simulink model "Control_scheme"  (R2020b)
settings: Solver=VariableStepAuto  StartTime=0.0  StopTime=200  RelTol=1e-3
values from neighbouring files (symbols this model uses):
  A = [5.11995503588 1 0 0 0 0 -11.4260465467 0 1 0 0 0 ... (36 elements, 6x6)]    [Estimated_Model.mat]
  Atrue = [-232280.917083 -1161395.21042 -696840.50125 -929117.855833 -232280.917083 -116142.271042 -247175.760189 -1235880.44867 -741527.985114 -988703.898712 -247175.851098 -123588.02214 ... (36 elements, 6x6)]    [barrassmodel2.mat]
  B = [1 0 0 0 0 0]    [Estimated_Model.mat]
  Btrue = [1 5 3 4 1 0.5]    [barrassmodel2.mat]
  C = [-6.48338492424e-05 0.00041393325507 -0.000527701144131 0.00055117489166 -0.000426728644373 0]    [Estimated_Model.mat]
  Ctrue = [2750000 -2204545.45455 32477272.7273 -15227272.7273 -18704545.4545 -19090909.0909]    [barrassmodel2.mat]
  D = 0    [Estimated_Model.mat]
  Dtrue = 0    [barrassmodel2.mat]
  Nbar = Nu+K*Nx    [LQE_LQR_par.m]    (also in demo.m)
  Ts = 1/fs    (= 0.01)    [BasicSim.m]    (also in IdentificationAlgorithm_best.m; LQE_LQR_par.m; demo.m)
undefined symbols (not defined in the file or in its folder): DiscIntNeverNeededParam, K, M
libraries: simulink x8
settings Model: Creator=Tripaskio  LastModifiedBy=renato

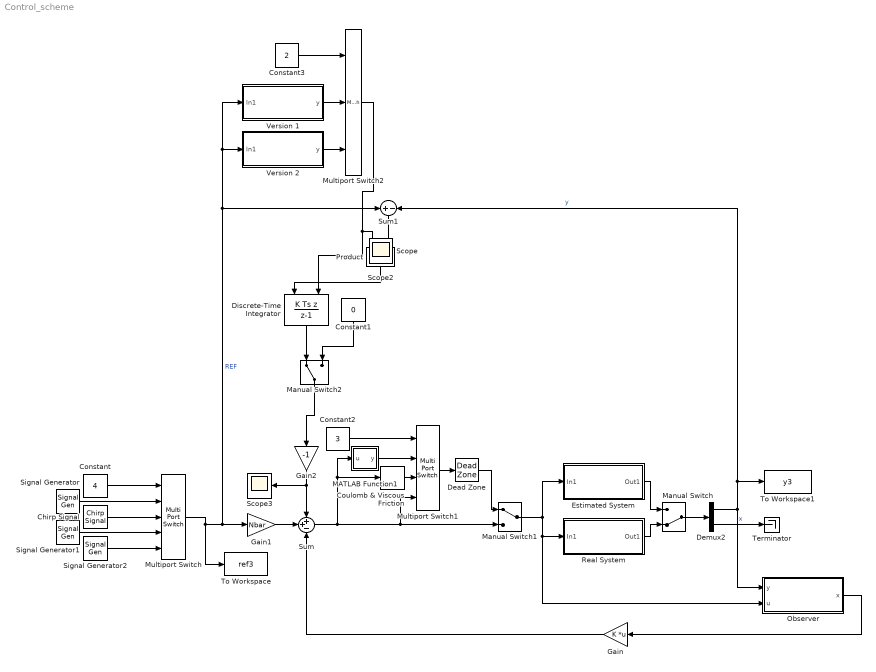
== system Control_scheme ==
  Chirp Signal : simulink/Sources/Chirp Signal  f1=0.01  T=200  f2=0.1
  Constant : Constant  Value=4
  Constant1 : Constant  Value=0
  Constant2 : Constant  Value=3
  Constant3 : Constant  Value=2
  Coulomb & Viscous Friction : simulink/Discontinuities/Coulomb & Viscous Friction  offset=[0.1]  gain=1
  Dead Zone : DeadZone  LowerValue=-0.1  UpperValue=0.1  SaturateOnIntegerOverflow=on
  Demux2 : Demux  Outputs=[1,6]
  Discrete-Time Integrator : DiscreteIntegrator  IntegratorMethod=Integration: Backward Euler  gainval=0.011  ExternalReset=either  SampleTime=-1  UpperSaturationLimit=10  LowerSaturationLimit=-10  ICPrevOutput=DiscIntNeverNeededParam  ICPrevScaledInput=DiscIntNeverNeededParam
  Estimated System : Subsystem
  Gain : Gain  Gain=K  Multiplication=Matrix(K*u)
  Gain1 : Gain  Gain=Nbar
  Gain2 : Gain  Gain=-1
  MATLAB Function1 : MATLAB Function  TreatAsAtomicUnit=on
  Manual Switch : ManualSwitch  CurrentSetting=0
  Manual Switch1 : ManualSwitch
  Manual Switch2 : ManualSwitch
  Multiport Switch : MultiPortSwitch  Inputs=4
  Multiport Switch1 : MultiPortSwitch
  Multiport Switch2 : MultiPortSwitch  Inputs=2
  Observer : Subsystem
  Product : Product
  Real System : Subsystem
  Scope3 : Scope
  Signal Generator : SignalGenerator  WaveForm=square  Amplitude=4  Frequency=0.1  Units=rad/sec
  Signal Generator1 : SignalGenerator  WaveForm=sawtooth  Amplitude=4  Frequency=0.11  Units=rad/sec
  Signal Generator2 : SignalGenerator  Amplitude=4  Frequency=0.15  Units=rad/sec
  Sum : Sum  Inputs=++-
  Sum1 : Sum  Inputs=+|-
  Terminator : Terminator
  To Workspace : ToWorkspace  VariableName=ref3  SaveFormat=Timeseries  SampleTime=-1
  To Workspace1 : ToWorkspace  VariableName=y3  SaveFormat=Timeseries  SampleTime=-1
  Version 1 : Subsystem
  Version 2 : Subsystem
  Scope : Scope
  Scope2 : Scope
  wires:
  Demux2/1 -> Observer/1(y), Sum1/2, To Workspace1/1  "y"
  Demux2/2 -> Terminator/1  "x"
  Observer/1(x) -> Gain/1
  Gain/1 -> Sum/3
  Gain1/1 -> Sum/2
  Signal Generator/1 -> Multiport Switch/2
  Manual Switch/1 -> Demux2/1
  Estimated System/1(Out1) -> Manual Switch/1
  Real System/1(Out1) -> Manual Switch/2
  Manual Switch1/1 -> Estimated System/1(In1), Observer/2(u), Real System/1(In1)
  Dead Zone/1 -> Manual Switch1/1
  Chirp Signal/1 -> Multiport Switch/3
  Signal Generator1/1 -> Multiport Switch/4
  Constant/1 -> Multiport Switch/1
  Discrete-Time Integrator/1 -> Manual Switch2/1
  Constant1/1 -> Manual Switch2/2
  Multiport Switch/1 -> To Workspace/1, Gain1/1, Sum1/1, Version 1/1(In1), Version 2/1(In1)  "REF"
  Signal Generator2/1 -> Multiport Switch/5
  Sum1/1 -> Product/2
  Product/1 -> Discrete-Time Integrator/1
  Manual Switch2/1 -> Gain2/1
  Gain2/1 -> Sum/1, Scope3/1
  Sum/1 -> MATLAB Function1/1(u), Coulomb & Viscous Friction/1, Multiport Switch1/4, Manual Switch1/2
  Coulomb & Viscous Friction/1 -> Multiport Switch1/3
  MATLAB Function1/1(y) -> Multiport Switch1/2
  Multiport Switch1/1 -> Dead Zone/1
  Constant2/1 -> Multiport Switch1/1
  Multiport Switch2/1 -> Discrete-Time Integrator/2, Product/1
  Version 2/1(y) -> Multiport Switch2/3
  Version 1/1(y) -> Multiport Switch2/2
  Constant3/1 -> Multiport Switch2/1

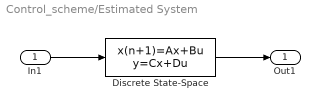
== system Control_scheme/Estimated System ==
  In1 : Inport
  Discrete State-Space : DiscreteStateSpace  A=A  B=B  C=[C ; eye(6)]  D=[D; 0;0;0;0;0;0]  SampleTime=0.01
  Out1 : Outport
  wires:
  In1/1 -> Discrete State-Space/1
  Discrete State-Space/1 -> Out1/1

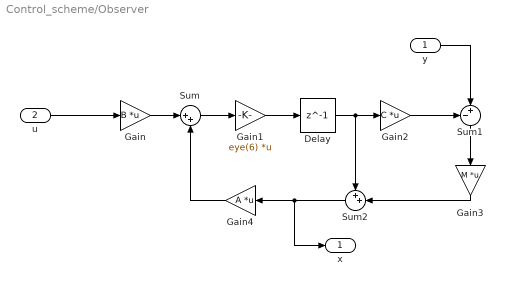
== system Control_scheme/Observer ==
  y : Inport
  u : Inport  Port=2
  Delay : Delay  DelayLength=1  SampleTime=Ts
  Gain : Gain  Gain=B  Multiplication=Matrix(K*u)
  Gain1 : Gain  Gain=eye(6)  Multiplication=Matrix(K*u)
  Gain2 : Gain  Gain=C  Multiplication=Matrix(K*u)
  Gain3 : Gain  Gain=M  Multiplication=Matrix(K*u)
  Gain4 : Gain  Gain=A  Multiplication=Matrix(K*u)
  Sum : Sum  Inputs=|++
  Sum1 : Sum  Inputs=-+|
  Sum2 : Sum  Inputs=++|
  x : Outport
  wires:
  u/1 -> Gain/1
  Gain/1 -> Sum/1
  Sum/1 -> Gain1/1
  Gain1/1 -> Delay/1
  Delay/1 -> Sum2/1, Gain2/1
  Gain2/1 -> Sum1/1
  y/1 -> Sum1/2
  Sum1/1 -> Gain3/1
  Gain4/1 -> Sum/2
  Sum2/1 -> x/1, Gain4/1
  Gain3/1 -> Sum2/2

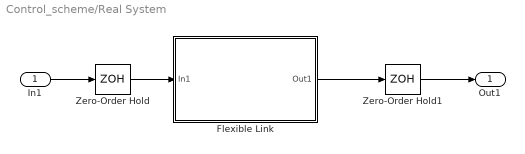
== system Control_scheme/Real System ==
  In1 : Inport
  Flexible Link : Subsystem
      mask Display: image('quanserlink.jpg')
  Zero-Order Hold : ZeroOrderHold  SampleTime=Ts
  Zero-Order Hold1 : ZeroOrderHold  SampleTime=Ts
  Out1 : Outport
  wires:
  In1/1 -> Zero-Order Hold/1
  Zero-Order Hold1/1 -> Out1/1
  Zero-Order Hold/1 -> Flexible Link/1(In1)
  Flexible Link/1(Out1) -> Zero-Order Hold1/1

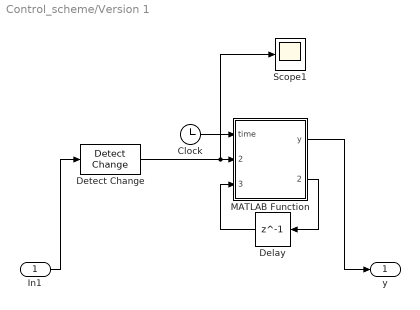
== system Control_scheme/Version 1 ==
  In1 : Inport
  Clock : Clock
  Delay : Delay  DelayLength=1
  Detect Change : simulink/Logic and Bit Operations/Detect Change  vinit=0  OutDataTypeStr=boolean
  MATLAB Function : MATLAB Function  TreatAsAtomicUnit=on
  Scope1 : Scope
  y : Outport
  wires:
  In1/1 -> Detect Change/1
  Clock/1 -> MATLAB Function/1(time)
  Detect Change/1 -> Scope1/1, MATLAB Function/2(change)
  MATLAB Function/1(y) -> y/1
  Delay/1 -> MATLAB Function/3("t_begin ")
  MATLAB Function/2(t_begin) -> Delay/1

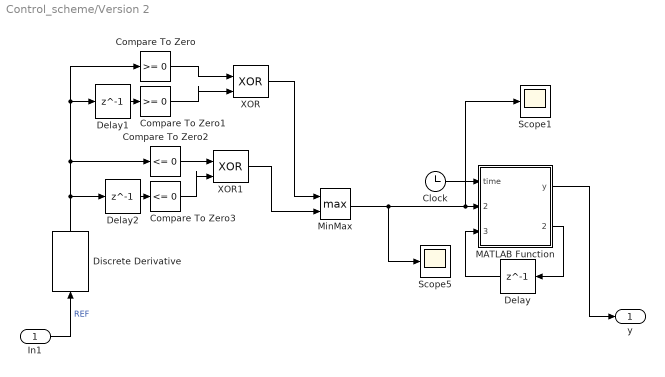
== system Control_scheme/Version 2 ==
  In1 : Inport
  Clock : Clock
  Compare To Zero : simulink/Logic and Bit Operations/Compare To Zero  relop=>=  OutDataTypeStr=boolean
  Compare To Zero1 : simulink/Logic and Bit Operations/Compare To Zero  relop=>=  OutDataTypeStr=boolean
  Compare To Zero2 : simulink/Logic and Bit Operations/Compare To Zero  relop=<=  OutDataTypeStr=boolean
  Compare To Zero3 : simulink/Logic and Bit Operations/Compare To Zero  relop=<=  OutDataTypeStr=boolean
  Delay : Delay  DelayLength=1
  Delay1 : Delay  DelayLength=1
  Delay2 : Delay  DelayLength=1
  Discrete Derivative : simulink/Discrete/Discrete Derivative  gainval=1.0  ICPrevScaledInput=0.0  OutMin=[]  OutMax=[]  OutDataType=fixdt(1, 16)  OutScaling=2^-10  DoSatur=off
  MATLAB Function : MATLAB Function  TreatAsAtomicUnit=on
  MinMax : MinMax  Function=max  Inputs=2
  Scope1 : Scope
  Scope5 : Scope
  XOR : Logic  Operator=XOR  IconShape=distinctive  AllPortsSameDT=off  OutDataTypeStr=boolean
  XOR1 : Logic  Operator=XOR  IconShape=distinctive  AllPortsSameDT=off  OutDataTypeStr=boolean
  y : Outport
  wires:
  MinMax/1 -> Scope1/1, MATLAB Function/2(change), Scope5/1
  XOR/1 -> MinMax/1
  In1/1 -> Discrete Derivative/1  "REF"
  Compare To Zero2/1 -> XOR1/1
  Delay1/1 -> Compare To Zero1/1
  Discrete Derivative/1 -> Delay2/1, Compare To Zero2/1, Delay1/1, Compare To Zero/1
  XOR1/1 -> MinMax/2
  Compare To Zero1/1 -> XOR/2
  Compare To Zero/1 -> XOR/1
  Delay2/1 -> Compare To Zero3/1
  MATLAB Function/2(t_begin) -> Delay/1
  Compare To Zero3/1 -> XOR1/2
  MATLAB Function/1(y) -> y/1
  Clock/1 -> MATLAB Function/1(time)
  Delay/1 -> MATLAB Function/3("t_begin ")

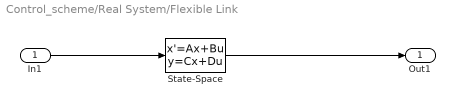
== system Control_scheme/Real System/Flexible Link ==
  In1 : Inport
  State-Space : StateSpace  A=Atrue  B=Btrue  C=Ctrue  D=Dtrue  InitialCondition=0
  Out1 : Outport
  wires:
  State-Space/1 -> Out1/1
  In1/1 -> State-Space/1

== matlab function Control_scheme/MATLAB Function1 ==
  data: u input; y output
function y = fcn(u)
    a=0.01;
    y=(exp(u/a)/(exp(u/a) + exp(-u/a)))*(u + 0.1) + ...
        (exp(-u/a)/(exp(u/a) + exp(-u/a)))*(u - 0.1);
end

== matlab function Control_scheme/Version 1/MATLAB Function ==
  data: time input; change input; y output; t_begin input; t_begin output
function [y,t_begin] = fcn(time,change,t_begin)
delta_t=5;
if time==0
    t_begin=time;
end
    if change==1
        t_begin=time;
    end
        
    if (time - t_begin)>delta_t
        y=1;
    else
        y=0;
    end
        
end

== matlab function Control_scheme/Version 2/MATLAB Function ==
  data: time input; change input; y output; t_begin input; t_begin output
function [y,t_begin] = fcn(time,change,t_begin)
delta_t=7;
if time==0
    t_begin=time;
end
    if change==1
        t_begin=time;
    end
        
    if (time - t_begin)>delta_t
        y=1;
    else
        y=0;
    end
        
end
